simulink model "gm_biquad_matlab"  (R2022a)
settings: Solver=VariableStepAuto  StartTime=0.0  StopTime=10.0  RelTol=1e-3
undefined symbols (not defined in the file): dfilt
libraries: dsparch4 x1
settings Model: Creator=Besic  LastModifiedBy=Besic
settings OptimizationCC: BlockReduction=off  ConditionallyExecuteInputs=off
settings DebuggingCC: InheritedTsInSrcMsg=none

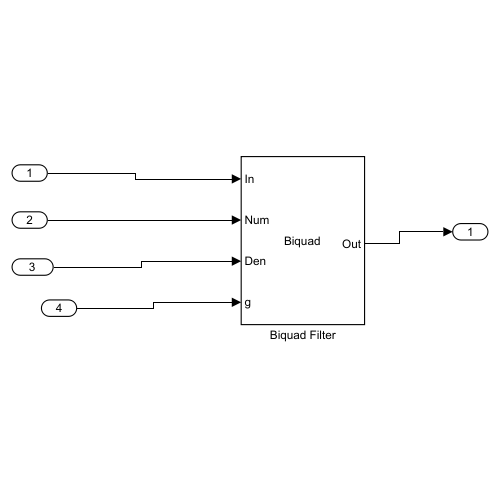
[thumbnail: Simulink's stored preview of the top-level diagram]
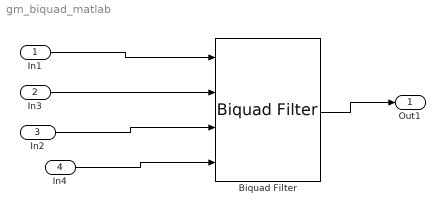
== system gm_biquad_matlab ==
  In1 : Inport  OutDataTypeStr=int16  PortDimensions=1  SampleTime=0.2
  In3 : Inport  Port=2  OutDataTypeStr=int16  PortDimensions=[3 1]  SampleTime=0.2
  In2 : Inport  Port=3  OutDataTypeStr=int16  PortDimensions=[2 1]  SampleTime=0.2
  In4 : Inport  Port=4  OutDataTypeStr=int16  PortDimensions=[1 2]  SampleTime=0.2
  Biquad Filter : dsparch4/Biquad Filter  FilterSource=Input port(s)  CoeffSource=Specify via dialog  FilterObject=dfilt.df2tsos([1 0.3 0.4],[1 0.1 0.2])  IIRFiltStruct=Direct form II transposed  BiQuadCoeffs="[0.035    0.035         0    1.0000   -0.9391         0]"  ScaleValues=1  IC=0  ICnum=0  ICden=0  a0Flag=Warning  optimizeScaleValues=on  ScaleValueMode=Specify via input port (g)  roundingMode=Floor  overflowMode=off  scaleValueFracLength=14  denProdOutputFracLength=30  denAccumFracLength=30  secondMemoryFracLength=15
  Out1 : Outport  OutDataTypeStr=int16  SampleTime=0.2
  wires:
  In1/1 -> Biquad Filter/1
  In3/1 -> Biquad Filter/2
  In2/1 -> Biquad Filter/3
  In4/1 -> Biquad Filter/4
  Biquad Filter/1 -> Out1/1
